simulink model "RAM_Design"  (R2025a)
settings: Solver=FixedStepDiscrete  StartTime=0.0  StopTime=10  FixedStep=1e-6  RelTol=1e-3
undefined symbols (not defined in the file): Bit_1, Bit_2, Bit_3, Bit_4, Bit_5, Bit_6, Bit_7, Bit_8
libraries: fl_lib x320, nesl_utility x136, simulink_extras x57
(part 1 of 5)
settings Model: PacingRate=0.050000  Creator=gerri  LastModifiedBy=gerri

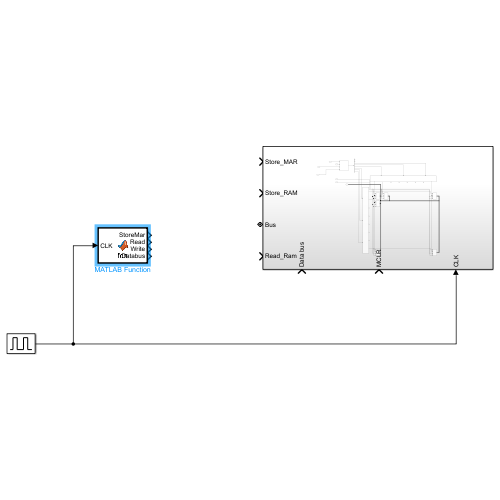
[thumbnail: Simulink's stored preview of the top-level diagram]
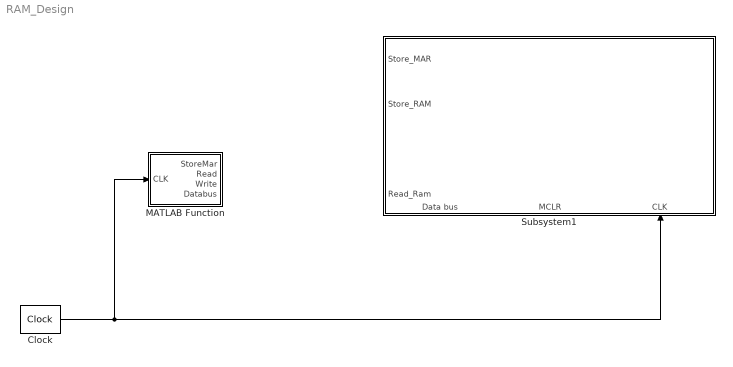
== system RAM_Design ==
  Clock : simulink_extras/Flip Flops/Clock  period=0.001
  MATLAB Function : MATLAB Function  TreatAsAtomicUnit=on
  Subsystem1 : Subsystem
      settings: PortSchema="{\"entries\":[{\"content\":{\"sides\":[{\"content\":{\"connectorIds\":[\"In1\",\"In2\",\"LConn1\",\"In3\"]},\"type\":\"ConnectorPlacement.EquallySpacedRectSide\",\"uuid\":\"fc099c56-c4b8-4508-a941-00bff1c84ffc\"},{\"content\":{\"side\":\"RIGHT\"},\"type\":\"ConnectorPlacement.EquallySpacedRectSide\",\"uuid\":\"202975a6-ae93-47c5-a757-f8e519a18074\"},{\"content\":{\"side\":\"TOP\"},\"type\":\"ConnectorPlacement.EquallySpacedRectSide\",\"uuid\":\"88b1988a-005b-4761-b740-e134c8683746\"},{\"content\":{\"connectorIds\":[\"In4\",\"In5\",\"In6\"],\"side\":\"BOTTOM\"},\"type\":\"ConnectorPlacement.EquallySpacedRectSide\",\"uuid\":\"5db4ec79-cfd7-4bc1-a90d-f6980e3bb618\"}]},\"type\":\"ConnectorPlacement.EquallySpacedConnector\",\"uuid\":\"bf959895-2947-4105-9e30-982428eecfc4\"}],\"packageUris\":[\"http://schema.mathworks.com/mf0/Connector/R2020b\"],\"version\":\"1.0\"}"
  wires:
  Clock/1 -> MATLAB Function/1(CLK), Subsystem1/6(CLK)

== system RAM_Design/Subsystem1 ==
  Store_MAR : Inport
  Store_RAM : Inport  Port=2
  Read_Ram : Inport  Port=3
  Data bus : Inport  Port=4
  MCLR : Inport  Port=5
  CLK : Inport  Port=6
  3*8_x : Subsystem
  3*8_y : Subsystem
  8Bit RAM 0 : Subsystem
  8Bit RAM 1 : Subsystem
  8Bit RAM 56 : Subsystem
  8Bit RAM 63 : Subsystem
  8Bit RAM 7 : Subsystem
  8Bit RAM 8 : Subsystem
  Demux : Demux  Outputs=8
  MAR : Subsystem
  Bus : PMIOPort  Side=Left
  wires:
  3*8_x/8(1/1/1) -> 8Bit RAM 7/1(x), 8Bit RAM 63/1(x)
  Demux/3 -> 3*8_y/3(Sel_C)
  3*8_x/1(0/0/0) -> 8Bit RAM 0/1(x), 8Bit RAM 8/1(x), 8Bit RAM 56/1(x)
  3*8_x/2(0/0/1) -> 8Bit RAM 1/1(x)
  3*8_y/1(0/0/0) -> 8Bit RAM 0/2(y), 8Bit RAM 1/2(y), 8Bit RAM 7/2(y)
  3*8_y/8(1/1/1) -> 8Bit RAM 63/2(y), 8Bit RAM 56/2(y)
  3*8_y/2(1/0/0) -> 8Bit RAM 8/2(y)
  Demux/4 -> 3*8_y/2(Sel_B)
  Demux/6 -> 3*8_x/1(Sel_A)
  Demux/7 -> 3*8_x/2(Sel_B)
  Demux/5 -> 3*8_y/1(Sel_A)
  MAR/1("Q Bus ") -> Demux/1
  Demux/8 -> 3*8_x/3(Sel_C)
  Store_RAM/1 -> 8Bit RAM 8/4(Store), 8Bit RAM 56/4(Store), 8Bit RAM 63/4(Store), 8Bit RAM 7/4(Store), 8Bit RAM 1/4(Store), 8Bit RAM 0/4(Store)
  CLK/1 -> MAR/3(CLK)
  Data bus/1 -> MAR/1(Data bus)
  Store_MAR/1 -> MAR/2(Store)
  MCLR/1 -> MAR/4(CLR)
  Read_Ram/1 -> 8Bit RAM 7/3(Enable), 8Bit RAM 1/3(Enable), 8Bit RAM 0/3(Enable), 8Bit RAM 56/3(Enable), 8Bit RAM 63/3(Enable), 8Bit RAM 8/3(Enable)
  connections:
  8Bit RAM 63/RConn1 -- 8Bit RAM 1/RConn1 -- 8Bit RAM 7/RConn1 -- 8Bit RAM 0/RConn1 -- Bus/RConn1 -- 8Bit RAM 8/RConn1 -- 8Bit RAM 56/RConn1

== system RAM_Design/Subsystem1/3*8_x ==
  note: A/B/C
  Sel_A : Inport
  Sel_B : Inport  Port=2
  Sel_C : Inport  Port=3
  AND{3..10} (8 alike) : Logic  Inputs=3  IconShape=distinctive  AllPortsSameDT=off  OutDataTypeStr=boolean
  NOT1 : Logic  Operator=NOT  IconShape=distinctive  AllPortsSameDT=off  OutDataTypeStr=boolean
  NOT2 : Logic  Operator=NOT  IconShape=distinctive  AllPortsSameDT=off  OutDataTypeStr=boolean
  NOT3 : Logic  Operator=NOT  IconShape=distinctive  AllPortsSameDT=off  OutDataTypeStr=boolean
  0/0/0 : Outport
  0/0/1 : Outport  Port=2
  0/1/0 : Outport  Port=3
  0/1/1 : Outport  Port=4
  1/0/0 : Outport  Port=5
  1/0/1 : Outport  Port=6
  1/1/0 : Outport  Port=7
  1/1/1 : Outport  Port=8
  wires:
  Sel_B/1 -> AND10/2, AND9/2, AND6/2, AND5/2, NOT2/1
  Sel_C/1 -> AND10/3, AND8/3, AND6/3, AND4/3, NOT3/1
  AND7/1 -> 1/0/0/1
  AND8/1 -> 1/0/1/1
  AND10/1 -> 1/1/1/1
  AND3/1 -> 0/0/0/1
  NOT1/1 -> AND6/1, AND5/1, AND4/1, AND3/1
  Sel_A/1 -> AND10/1, AND9/1, AND8/1, AND7/1, NOT1/1
  NOT3/1 -> AND9/3, AND7/3, AND5/3, AND3/3
  AND5/1 -> 0/1/0/1
  NOT2/1 -> AND4/2, AND7/2, AND8/2, AND3/2
  AND9/1 -> 1/1/0/1
  AND6/1 -> 0/1/1/1
  AND4/1 -> 0/0/1/1

== system RAM_Design/Subsystem1/3*8_y ==
  note: A/B/C
  Sel_A : Inport
  Sel_B : Inport  Port=2
  Sel_C : Inport  Port=3
  AND{3..10} (8 alike) : Logic  Inputs=3  IconShape=distinctive  AllPortsSameDT=off  OutDataTypeStr=boolean
  NOT1 : Logic  Operator=NOT  IconShape=distinctive  AllPortsSameDT=off  OutDataTypeStr=boolean
  NOT2 : Logic  Operator=NOT  IconShape=distinctive  AllPortsSameDT=off  OutDataTypeStr=boolean
  NOT3 : Logic  Operator=NOT  IconShape=distinctive  AllPortsSameDT=off  OutDataTypeStr=boolean
  0/0/0 : Outport
  1/0/0 : Outport  Port=2
  0/1/0 : Outport  Port=3
  1/1/0 : Outport  Port=4
  0/0/1 : Outport  Port=5
  1/0/1 : Outport  Port=6
  0/1/1 : Outport  Port=7
  1/1/1 : Outport  Port=8
  wires:
  Sel_B/1 -> AND10/2, AND9/2, AND6/2, AND5/2, NOT2/1
  Sel_C/1 -> AND10/3, AND8/3, AND6/3, AND4/3, NOT3/1
  AND7/1 -> 1/0/0/1
  AND8/1 -> 1/0/1/1
  AND10/1 -> 1/1/1/1
  AND3/1 -> 0/0/0/1
  NOT1/1 -> AND6/1, AND5/1, AND4/1, AND3/1
  Sel_A/1 -> AND10/1, AND9/1, AND8/1, AND7/1, NOT1/1
  NOT3/1 -> AND9/3, AND7/3, AND5/3, AND3/3
  AND5/1 -> 0/1/0/1
  NOT2/1 -> AND4/2, AND7/2, AND8/2, AND3/2
  AND9/1 -> 1/1/0/1
  AND6/1 -> 0/1/1/1
  AND4/1 -> 0/0/1/1

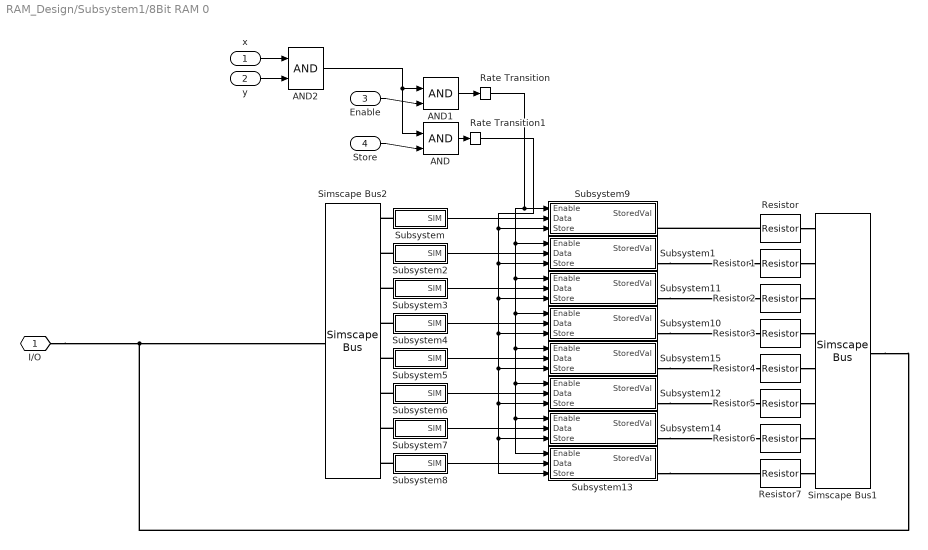
== system RAM_Design/Subsystem1/8Bit RAM 0 ==
  x : Inport
  y : Inport  Port=2
  Enable : Inport  Port=3
  Store : Inport  Port=4
  AND : Logic  IconShape=distinctive  AllPortsSameDT=off  OutDataTypeStr=boolean
  AND1 : Logic  IconShape=distinctive  AllPortsSameDT=off  OutDataTypeStr=boolean
  AND2 : Logic  IconShape=distinctive  AllPortsSameDT=off  OutDataTypeStr=boolean
  Rate Transition : RateTransition
  Rate Transition1 : RateTransition
  Resistor{,1..7} (8 alike) : fl_lib/Electrical/Electrical Elements/Resistor  R=1 Ohm  i_specify=off  i_priority=None  i=0 A  i_nominal_specify=off  i_nominal_value=1  i_nominal_unit=A  v_specify=off  v_priority=None  v=0 V  v_nominal_specify=off  v_nominal_value=1  v_nominal_unit=V
  Simscape Bus1 : SimscapeBus  HierarchyStrings=Bit_8;Bit_7;Bit_6;Bit_5;Bit_4;Bit_3;Bit_2;Bit_1
  Simscape Bus2 : SimscapeBus  HierarchyStrings=Bit_8;Bit_7;Bit_6;Bit_5;Bit_4;Bit_3;Bit_2;Bit_1
  Subsystem : Subsystem
  Subsystem1 : Subsystem
  Subsystem10 : Subsystem
  Subsystem11 : Subsystem
  Subsystem12 : Subsystem
  Subsystem13 : Subsystem
  Subsystem14 : Subsystem
  Subsystem15 : Subsystem
  Subsystem2 : Subsystem
  Subsystem3 : Subsystem
  Subsystem4 : Subsystem
  Subsystem5 : Subsystem
  Subsystem6 : Subsystem
  Subsystem7 : Subsystem
  Subsystem8 : Subsystem
  Subsystem9 : Subsystem
  I/O : PMIOPort  Side=Right
  wires:
  Enable/1 -> AND1/2
  Store/1 -> AND/2
  AND2/1 -> AND/1, AND1/1
  x/1 -> AND2/1
  y/1 -> AND2/2
  Subsystem/1(SIM) -> Subsystem9/2(Data)
  Subsystem2/1(SIM) -> Subsystem1/2(Data)
  Subsystem3/1(SIM) -> Subsystem11/2(Data)
  Subsystem4/1(SIM) -> Subsystem10/2(Data)
  Rate Transition1/1 -> Subsystem1/3(Store), Subsystem11/3(Store), Subsystem10/3(Store), Subsystem15/3(Store), Subsystem12/3(Store), Subsystem14/3(Store), Subsystem13/3(Store), Subsystem9/3(Store)
  AND1/1 -> Rate Transition/1
  Subsystem8/1(SIM) -> Subsystem13/2(Data)
  Subsystem7/1(SIM) -> Subsystem14/2(Data)
  Subsystem6/1(SIM) -> Subsystem12/2(Data)
  Subsystem5/1(SIM) -> Subsystem15/2(Data)
  Rate Transition/1 -> Subsystem1/1(Enable), Subsystem11/1(Enable), Subsystem10/1(Enable), Subsystem15/1(Enable), Subsystem12/1(Enable), Subsystem13/1(Enable), Subsystem14/1(Enable), Subsystem9/1(Enable)
  AND/1 -> Rate Transition1/1
  connections:
  I/O/RConn1 -- Simscape Bus1/RConn1 -- Simscape Bus2/RConn1
  Subsystem/LConn1 -- Simscape Bus2/LConn1
  Subsystem2/LConn1 -- Simscape Bus2/LConn2
  Subsystem4/LConn1 -- Simscape Bus2/LConn4
  Subsystem8/LConn1 -- Simscape Bus2/LConn8
  Subsystem6/LConn1 -- Simscape Bus2/LConn6
  Subsystem5/LConn1 -- Simscape Bus2/LConn5
  Subsystem7/LConn1 -- Simscape Bus2/LConn7
  Subsystem3/LConn1 -- Simscape Bus2/LConn3
  Resistor/RConn1 -- Simscape Bus1/LConn1
  Resistor/LConn1 -- Subsystem9/RConn1
  Subsystem1/RConn1 -- Resistor1/LConn1
  Resistor1/RConn1 -- Simscape Bus1/LConn2
  Subsystem10/RConn1 -- Resistor3/LConn1
  Subsystem11/RConn1 -- Resistor2/LConn1
  Resistor3/RConn1 -- Simscape Bus1/LConn4
  Resistor7/RConn1 -- Simscape Bus1/LConn8
  Resistor6/RConn1 -- Simscape Bus1/LConn7
  Resistor5/RConn1 -- Simscape Bus1/LConn6
  Resistor4/RConn1 -- Simscape Bus1/LConn5
  Resistor2/RConn1 -- Simscape Bus1/LConn3
  Subsystem15/RConn1 -- Resistor4/LConn1
  Subsystem12/RConn1 -- Resistor5/LConn1
  Subsystem14/RConn1 -- Resistor6/LConn1
  Subsystem13/RConn1 -- Resistor7/LConn1

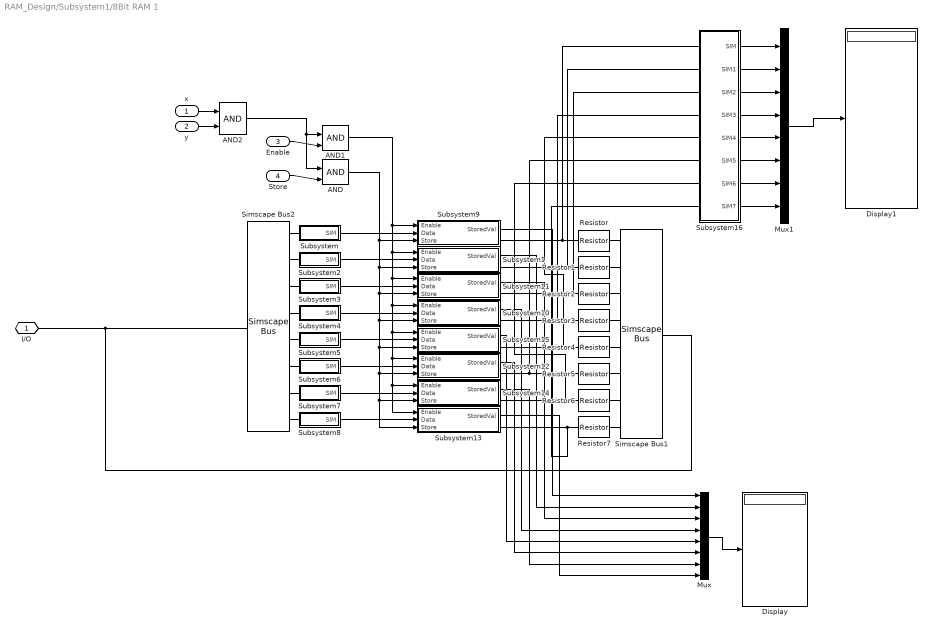
== system RAM_Design/Subsystem1/8Bit RAM 1 ==
  x : Inport
  y : Inport  Port=2
  Enable : Inport  Port=3
  Store : Inport  Port=4
  AND : Logic  IconShape=distinctive  AllPortsSameDT=off  OutDataTypeStr=boolean
  AND1 : Logic  IconShape=distinctive  AllPortsSameDT=off  OutDataTypeStr=boolean
  AND2 : Logic  IconShape=distinctive  AllPortsSameDT=off  OutDataTypeStr=boolean
  Display : Display
  Display1 : Display
  Mux : Mux  Inputs=8
  Mux1 : Mux  Inputs=8
  Resistor{,1..7} (8 alike) : fl_lib/Electrical/Electrical Elements/Resistor  R=1 Ohm  i_specify=off  i_priority=None  i=0 A  i_nominal_specify=off  i_nominal_value=1  i_nominal_unit=A  v_specify=off  v_priority=None  v=0 V  v_nominal_specify=off  v_nominal_value=1  v_nominal_unit=V
  Simscape Bus1 : SimscapeBus  HierarchyStrings=Bit_8;Bit_7;Bit_6;Bit_5;Bit_4;Bit_3;Bit_2;Bit_1
  Simscape Bus2 : SimscapeBus  HierarchyStrings=Bit_8;Bit_7;Bit_6;Bit_5;Bit_4;Bit_3;Bit_2;Bit_1
  Subsystem : Subsystem
  Subsystem1 : Subsystem
  Subsystem10 : Subsystem
  Subsystem11 : Subsystem
  Subsystem12 : Subsystem
  Subsystem13 : Subsystem
  Subsystem14 : Subsystem
  Subsystem15 : Subsystem
  Subsystem16 : Subsystem
  Subsystem2 : Subsystem
  Subsystem3 : Subsystem
  Subsystem4 : Subsystem
  Subsystem5 : Subsystem
  Subsystem6 : Subsystem
  Subsystem7 : Subsystem
  Subsystem8 : Subsystem
  Subsystem9 : Subsystem
  I/O : PMIOPort  Side=Right
  wires:
  Enable/1 -> AND1/2
  Store/1 -> AND/2
  AND2/1 -> AND/1, AND1/1
  x/1 -> AND2/1
  y/1 -> AND2/2
  Subsystem/1(SIM) -> Subsystem9/2(Data)
  Subsystem2/1(SIM) -> Subsystem1/2(Data)
  Subsystem3/1(SIM) -> Subsystem11/2(Data)
  Subsystem4/1(SIM) -> Subsystem10/2(Data)
  AND/1 -> Subsystem1/3(Store), Subsystem11/3(Store), Subsystem10/3(Store), Subsystem15/3(Store), Subsystem12/3(Store), Subsystem14/3(Store), Subsystem13/3(Store), Subsystem9/3(Store)
  AND1/1 -> Subsystem1/1(Enable), Subsystem11/1(Enable), Subsystem10/1(Enable), Subsystem15/1(Enable), Subsystem12/1(Enable), Subsystem13/1(Enable), Subsystem14/1(Enable), Subsystem9/1(Enable)
  Subsystem8/1(SIM) -> Subsystem13/2(Data)
  Subsystem7/1(SIM) -> Subsystem14/2(Data)
  Subsystem6/1(SIM) -> Subsystem12/2(Data)
  Subsystem5/1(SIM) -> Subsystem15/2(Data)
  Mux/1 -> Display/1
  Subsystem9/1(StoredVal) -> Mux/1
  Subsystem1/1(StoredVal) -> Mux/2
  Subsystem11/1(StoredVal) -> Mux/3
  Subsystem10/1(StoredVal) -> Mux/4
  Subsystem15/1(StoredVal) -> Mux/5
  Subsystem12/1(StoredVal) -> Mux/6
  Subsystem14/1(StoredVal) -> Mux/7
  Subsystem13/1(StoredVal) -> Mux/8
  Subsystem16/8(SIM7) -> Mux1/8
  Subsystem16/3(SIM2) -> Mux1/3
  Subsystem16/7(SIM6) -> Mux1/7
  Subsystem16/4(SIM3) -> Mux1/4
  Subsystem16/6(SIM5) -> Mux1/6
  Subsystem16/1(SIM) -> Mux1/1
  Subsystem16/5(SIM4) -> Mux1/5
  Subsystem16/2(SIM1) -> Mux1/2
  Mux1/1 -> Display1/1
  connections:
  I/O/RConn1 -- Simscape Bus1/RConn1 -- Simscape Bus2/RConn1
  Subsystem/LConn1 -- Simscape Bus2/LConn1
  Subsystem2/LConn1 -- Simscape Bus2/LConn2
  Subsystem4/LConn1 -- Simscape Bus2/LConn4
  Subsystem8/LConn1 -- Simscape Bus2/LConn8
  Subsystem6/LConn1 -- Simscape Bus2/LConn6
  Subsystem5/LConn1 -- Simscape Bus2/LConn5
  Subsystem7/LConn1 -- Simscape Bus2/LConn7
  Subsystem3/LConn1 -- Simscape Bus2/LConn3
  Resistor/RConn1 -- Simscape Bus1/LConn1
  Resistor/LConn1 -- Subsystem16/LConn1 -- Subsystem9/RConn1
  Resistor1/LConn1 -- Subsystem1/RConn1 -- Subsystem16/LConn2
  Resistor1/RConn1 -- Simscape Bus1/LConn2
  Resistor3/LConn1 -- Subsystem10/RConn1 -- Subsystem16/LConn4
  Resistor2/LConn1 -- Subsystem11/RConn1 -- Subsystem16/LConn3
  Resistor3/RConn1 -- Simscape Bus1/LConn4
  Resistor7/RConn1 -- Simscape Bus1/LConn8
  Resistor6/RConn1 -- Simscape Bus1/LConn7
  Resistor5/RConn1 -- Simscape Bus1/LConn6
  Resistor4/RConn1 -- Simscape Bus1/LConn5
  Resistor2/RConn1 -- Simscape Bus1/LConn3
  Resistor4/LConn1 -- Subsystem15/RConn1 -- Subsystem16/LConn5
  Resistor5/LConn1 -- Subsystem12/RConn1 -- Subsystem16/LConn6
  Resistor6/LConn1 -- Subsystem14/RConn1 -- Subsystem16/LConn7
  Resistor7/LConn1 -- Subsystem13/RConn1 -- Subsystem16/LConn8

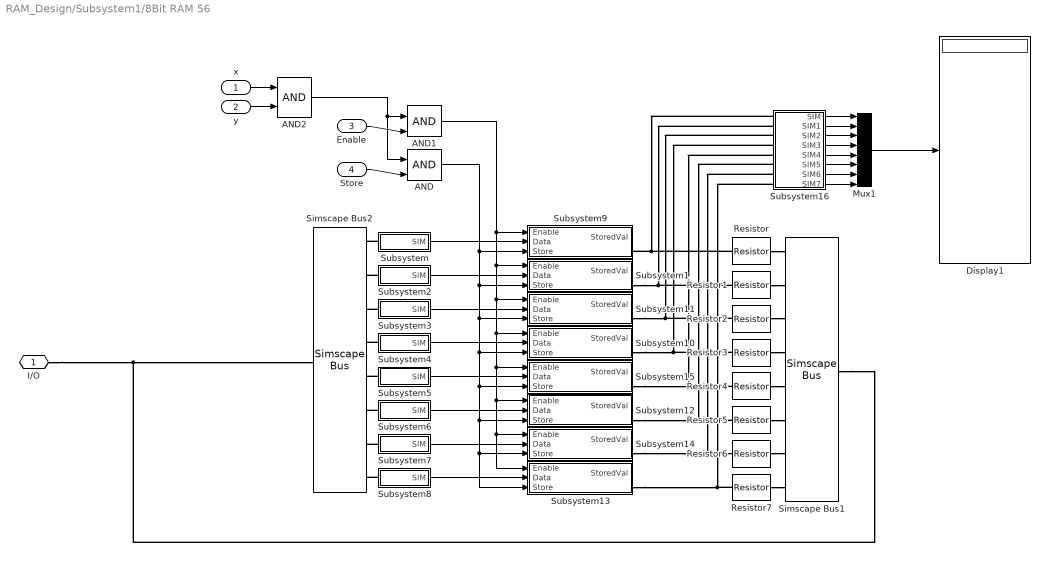
== system RAM_Design/Subsystem1/8Bit RAM 56 ==
  x : Inport
  y : Inport  Port=2
  Enable : Inport  Port=3
  Store : Inport  Port=4
  AND : Logic  IconShape=distinctive  AllPortsSameDT=off  OutDataTypeStr=boolean
  AND1 : Logic  IconShape=distinctive  AllPortsSameDT=off  OutDataTypeStr=boolean
  AND2 : Logic  IconShape=distinctive  AllPortsSameDT=off  OutDataTypeStr=boolean
  Display1 : Display
  Mux1 : Mux  Inputs=8
  Resistor{,1..7} (8 alike) : fl_lib/Electrical/Electrical Elements/Resistor  R=1 Ohm  i_specify=off  i_priority=None  i=0 A  i_nominal_specify=off  i_nominal_value=1  i_nominal_unit=A  v_specify=off  v_priority=None  v=0 V  v_nominal_specify=off  v_nominal_value=1  v_nominal_unit=V
  Simscape Bus1 : SimscapeBus  HierarchyStrings=Bit_8;Bit_7;Bit_6;Bit_5;Bit_4;Bit_3;Bit_2;Bit_1
  Simscape Bus2 : SimscapeBus  HierarchyStrings=Bit_8;Bit_7;Bit_6;Bit_5;Bit_4;Bit_3;Bit_2;Bit_1
  Subsystem : Subsystem
  Subsystem1 : Subsystem
  Subsystem10 : Subsystem
  Subsystem11 : Subsystem
  Subsystem12 : Subsystem
  Subsystem13 : Subsystem
  Subsystem14 : Subsystem
  Subsystem15 : Subsystem
  Subsystem16 : Subsystem
  Subsystem2 : Subsystem
  Subsystem3 : Subsystem
  Subsystem4 : Subsystem
  Subsystem5 : Subsystem
  Subsystem6 : Subsystem
  Subsystem7 : Subsystem
  Subsystem8 : Subsystem
  Subsystem9 : Subsystem
  I/O : PMIOPort  Side=Right
  wires:
  Enable/1 -> AND1/2
  Store/1 -> AND/2
  AND2/1 -> AND/1, AND1/1
  x/1 -> AND2/1
  y/1 -> AND2/2
  Subsystem/1(SIM) -> Subsystem9/2(Data)
  Subsystem2/1(SIM) -> Subsystem1/2(Data)
  Subsystem3/1(SIM) -> Subsystem11/2(Data)
  Subsystem4/1(SIM) -> Subsystem10/2(Data)
  AND/1 -> Subsystem1/3(Store), Subsystem11/3(Store), Subsystem10/3(Store), Subsystem15/3(Store), Subsystem12/3(Store), Subsystem14/3(Store), Subsystem13/3(Store), Subsystem9/3(Store)
  AND1/1 -> Subsystem1/1(Enable), Subsystem11/1(Enable), Subsystem10/1(Enable), Subsystem15/1(Enable), Subsystem12/1(Enable), Subsystem13/1(Enable), Subsystem14/1(Enable), Subsystem9/1(Enable)
  Subsystem8/1(SIM) -> Subsystem13/2(Data)
  Subsystem7/1(SIM) -> Subsystem14/2(Data)
  Subsystem6/1(SIM) -> Subsystem12/2(Data)
  Subsystem5/1(SIM) -> Subsystem15/2(Data)
  Subsystem16/8(SIM7) -> Mux1/8
  Subsystem16/3(SIM2) -> Mux1/3
  Subsystem16/7(SIM6) -> Mux1/7
  Subsystem16/4(SIM3) -> Mux1/4
  Subsystem16/6(SIM5) -> Mux1/6
  Subsystem16/1(SIM) -> Mux1/1
  Subsystem16/5(SIM4) -> Mux1/5
  Subsystem16/2(SIM1) -> Mux1/2
  Mux1/1 -> Display1/1
  connections:
  I/O/RConn1 -- Simscape Bus1/RConn1 -- Simscape Bus2/RConn1
  Subsystem/LConn1 -- Simscape Bus2/LConn1
  Subsystem2/LConn1 -- Simscape Bus2/LConn2
  Subsystem4/LConn1 -- Simscape Bus2/LConn4
  Subsystem8/LConn1 -- Simscape Bus2/LConn8
  Subsystem6/LConn1 -- Simscape Bus2/LConn6
  Subsystem5/LConn1 -- Simscape Bus2/LConn5
  Subsystem7/LConn1 -- Simscape Bus2/LConn7
  Subsystem3/LConn1 -- Simscape Bus2/LConn3
  Resistor/RConn1 -- Simscape Bus1/LConn1
  Subsystem16/LConn1 -- Resistor/LConn1 -- Subsystem9/RConn1
  Resistor1/LConn1 -- Subsystem1/RConn1 -- Subsystem16/LConn2
  Resistor1/RConn1 -- Simscape Bus1/LConn2
  Resistor3/LConn1 -- Subsystem10/RConn1 -- Subsystem16/LConn4
  Resistor2/LConn1 -- Subsystem11/RConn1 -- Subsystem16/LConn3
  Resistor3/RConn1 -- Simscape Bus1/LConn4
  Resistor7/RConn1 -- Simscape Bus1/LConn8
  Resistor6/RConn1 -- Simscape Bus1/LConn7
  Resistor5/RConn1 -- Simscape Bus1/LConn6
  Resistor4/RConn1 -- Simscape Bus1/LConn5
  Resistor2/RConn1 -- Simscape Bus1/LConn3
  Resistor4/LConn1 -- Subsystem15/RConn1 -- Subsystem16/LConn5
  Resistor5/LConn1 -- Subsystem12/RConn1 -- Subsystem16/LConn6
  Subsystem14/RConn1 -- Resistor6/LConn1 -- Subsystem16/LConn7
  Subsystem13/RConn1 -- Resistor7/LConn1 -- Subsystem16/LConn8

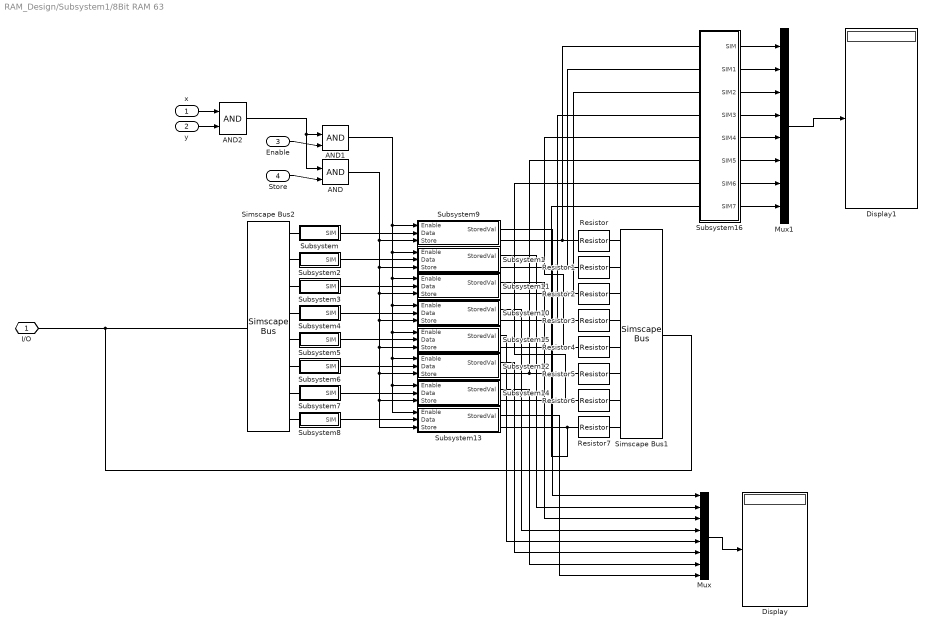
== system RAM_Design/Subsystem1/8Bit RAM 63 ==
  x : Inport
  y : Inport  Port=2
  Enable : Inport  Port=3
  Store : Inport  Port=4
  AND : Logic  IconShape=distinctive  AllPortsSameDT=off  OutDataTypeStr=boolean
  AND1 : Logic  IconShape=distinctive  AllPortsSameDT=off  OutDataTypeStr=boolean
  AND2 : Logic  IconShape=distinctive  AllPortsSameDT=off  OutDataTypeStr=boolean
  Display : Display
  Display1 : Display
  Mux : Mux  Inputs=8
  Mux1 : Mux  Inputs=8
  Resistor{,1..7} (8 alike) : fl_lib/Electrical/Electrical Elements/Resistor  R=1 Ohm  i_specify=off  i_priority=None  i=0 A  i_nominal_specify=off  i_nominal_value=1  i_nominal_unit=A  v_specify=off  v_priority=None  v=0 V  v_nominal_specify=off  v_nominal_value=1  v_nominal_unit=V
  Simscape Bus1 : SimscapeBus  HierarchyStrings=Bit_8;Bit_7;Bit_6;Bit_5;Bit_4;Bit_3;Bit_2;Bit_1
  Simscape Bus2 : SimscapeBus  HierarchyStrings=Bit_8;Bit_7;Bit_6;Bit_5;Bit_4;Bit_3;Bit_2;Bit_1
  Subsystem : Subsystem
  Subsystem1 : Subsystem
  Subsystem10 : Subsystem
  Subsystem11 : Subsystem
  Subsystem12 : Subsystem
  Subsystem13 : Subsystem
  Subsystem14 : Subsystem
  Subsystem15 : Subsystem
  Subsystem16 : Subsystem
  Subsystem2 : Subsystem
  Subsystem3 : Subsystem
  Subsystem4 : Subsystem
  Subsystem5 : Subsystem
  Subsystem6 : Subsystem
  Subsystem7 : Subsystem
  Subsystem8 : Subsystem
  Subsystem9 : Subsystem
  I/O : PMIOPort  Side=Right
  wires:
  Enable/1 -> AND1/2
  Store/1 -> AND/2
  AND2/1 -> AND/1, AND1/1
  x/1 -> AND2/1
  y/1 -> AND2/2
  Subsystem/1(SIM) -> Subsystem9/2(Data)
  Subsystem2/1(SIM) -> Subsystem1/2(Data)
  Subsystem3/1(SIM) -> Subsystem11/2(Data)
  Subsystem4/1(SIM) -> Subsystem10/2(Data)
  AND/1 -> Subsystem1/3(Store), Subsystem11/3(Store), Subsystem10/3(Store), Subsystem15/3(Store), Subsystem12/3(Store), Subsystem14/3(Store), Subsystem13/3(Store), Subsystem9/3(Store)
  AND1/1 -> Subsystem1/1(Enable), Subsystem11/1(Enable), Subsystem10/1(Enable), Subsystem15/1(Enable), Subsystem12/1(Enable), Subsystem13/1(Enable), Subsystem14/1(Enable), Subsystem9/1(Enable)
  Subsystem8/1(SIM) -> Subsystem13/2(Data)
  Subsystem7/1(SIM) -> Subsystem14/2(Data)
  Subsystem6/1(SIM) -> Subsystem12/2(Data)
  Subsystem5/1(SIM) -> Subsystem15/2(Data)
  Mux/1 -> Display/1
  Subsystem9/1(StoredVal) -> Mux/1
  Subsystem1/1(StoredVal) -> Mux/2
  Subsystem11/1(StoredVal) -> Mux/3
  Subsystem10/1(StoredVal) -> Mux/4
  Subsystem15/1(StoredVal) -> Mux/5
  Subsystem12/1(StoredVal) -> Mux/6
  Subsystem14/1(StoredVal) -> Mux/7
  Subsystem13/1(StoredVal) -> Mux/8
  Subsystem16/8(SIM7) -> Mux1/8
  Subsystem16/3(SIM2) -> Mux1/3
  Subsystem16/7(SIM6) -> Mux1/7
  Subsystem16/4(SIM3) -> Mux1/4
  Subsystem16/6(SIM5) -> Mux1/6
  Subsystem16/1(SIM) -> Mux1/1
  Subsystem16/5(SIM4) -> Mux1/5
  Subsystem16/2(SIM1) -> Mux1/2
  Mux1/1 -> Display1/1
  connections:
  I/O/RConn1 -- Simscape Bus1/RConn1 -- Simscape Bus2/RConn1
  Subsystem/LConn1 -- Simscape Bus2/LConn1
  Subsystem2/LConn1 -- Simscape Bus2/LConn2
  Subsystem4/LConn1 -- Simscape Bus2/LConn4
  Subsystem8/LConn1 -- Simscape Bus2/LConn8
  Subsystem6/LConn1 -- Simscape Bus2/LConn6
  Subsystem5/LConn1 -- Simscape Bus2/LConn5
  Subsystem7/LConn1 -- Simscape Bus2/LConn7
  Subsystem3/LConn1 -- Simscape Bus2/LConn3
  Resistor/RConn1 -- Simscape Bus1/LConn1
  Resistor/LConn1 -- Subsystem16/LConn1 -- Subsystem9/RConn1
  Resistor1/LConn1 -- Subsystem1/RConn1 -- Subsystem16/LConn2
  Resistor1/RConn1 -- Simscape Bus1/LConn2
  Resistor3/LConn1 -- Subsystem10/RConn1 -- Subsystem16/LConn4
  Resistor2/LConn1 -- Subsystem11/RConn1 -- Subsystem16/LConn3
  Resistor3/RConn1 -- Simscape Bus1/LConn4
  Resistor7/RConn1 -- Simscape Bus1/LConn8
  Resistor6/RConn1 -- Simscape Bus1/LConn7
  Resistor5/RConn1 -- Simscape Bus1/LConn6
  Resistor4/RConn1 -- Simscape Bus1/LConn5
  Resistor2/RConn1 -- Simscape Bus1/LConn3
  Resistor4/LConn1 -- Subsystem15/RConn1 -- Subsystem16/LConn5
  Resistor5/LConn1 -- Subsystem12/RConn1 -- Subsystem16/LConn6
  Resistor6/LConn1 -- Subsystem14/RConn1 -- Subsystem16/LConn7
  Resistor7/LConn1 -- Subsystem13/RConn1 -- Subsystem16/LConn8

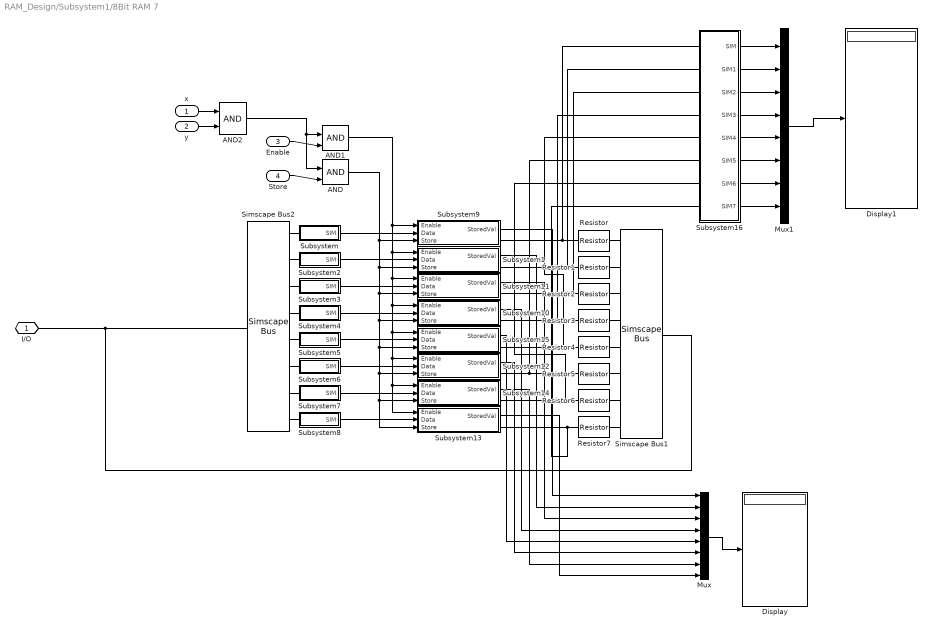
== system RAM_Design/Subsystem1/8Bit RAM 7 ==
  x : Inport
  y : Inport  Port=2
  Enable : Inport  Port=3
  Store : Inport  Port=4
  AND : Logic  IconShape=distinctive  AllPortsSameDT=off  OutDataTypeStr=boolean
  AND1 : Logic  IconShape=distinctive  AllPortsSameDT=off  OutDataTypeStr=boolean
  AND2 : Logic  IconShape=distinctive  AllPortsSameDT=off  OutDataTypeStr=boolean
  Display : Display
  Display1 : Display
  Mux : Mux  Inputs=8
  Mux1 : Mux  Inputs=8
  Resistor{,1..7} (8 alike) : fl_lib/Electrical/Electrical Elements/Resistor  R=1 Ohm  i_specify=off  i_priority=None  i=0 A  i_nominal_specify=off  i_nominal_value=1  i_nominal_unit=A  v_specify=off  v_priority=None  v=0 V  v_nominal_specify=off  v_nominal_value=1  v_nominal_unit=V
  Simscape Bus1 : SimscapeBus  HierarchyStrings=Bit_8;Bit_7;Bit_6;Bit_5;Bit_4;Bit_3;Bit_2;Bit_1
  Simscape Bus2 : SimscapeBus  HierarchyStrings=Bit_8;Bit_7;Bit_6;Bit_5;Bit_4;Bit_3;Bit_2;Bit_1
  Subsystem : Subsystem
  Subsystem1 : Subsystem
  Subsystem10 : Subsystem
  Subsystem11 : Subsystem
  Subsystem12 : Subsystem
  Subsystem13 : Subsystem
  Subsystem14 : Subsystem
  Subsystem15 : Subsystem
  Subsystem16 : Subsystem
  Subsystem2 : Subsystem
  Subsystem3 : Subsystem
  Subsystem4 : Subsystem
  Subsystem5 : Subsystem
  Subsystem6 : Subsystem
  Subsystem7 : Subsystem
  Subsystem8 : Subsystem
  Subsystem9 : Subsystem
  I/O : PMIOPort  Side=Right
  wires:
  Enable/1 -> AND1/2
  Store/1 -> AND/2
  AND2/1 -> AND/1, AND1/1
  x/1 -> AND2/1
  y/1 -> AND2/2
  Subsystem/1(SIM) -> Subsystem9/2(Data)
  Subsystem2/1(SIM) -> Subsystem1/2(Data)
  Subsystem3/1(SIM) -> Subsystem11/2(Data)
  Subsystem4/1(SIM) -> Subsystem10/2(Data)
  AND/1 -> Subsystem1/3(Store), Subsystem11/3(Store), Subsystem10/3(Store), Subsystem15/3(Store), Subsystem12/3(Store), Subsystem14/3(Store), Subsystem13/3(Store), Subsystem9/3(Store)
  AND1/1 -> Subsystem1/1(Enable), Subsystem11/1(Enable), Subsystem10/1(Enable), Subsystem15/1(Enable), Subsystem12/1(Enable), Subsystem13/1(Enable), Subsystem14/1(Enable), Subsystem9/1(Enable)
  Subsystem8/1(SIM) -> Subsystem13/2(Data)
  Subsystem7/1(SIM) -> Subsystem14/2(Data)
  Subsystem6/1(SIM) -> Subsystem12/2(Data)
  Subsystem5/1(SIM) -> Subsystem15/2(Data)
  Mux/1 -> Display/1
  Subsystem9/1(StoredVal) -> Mux/1
  Subsystem1/1(StoredVal) -> Mux/2
  Subsystem11/1(StoredVal) -> Mux/3
  Subsystem10/1(StoredVal) -> Mux/4
  Subsystem15/1(StoredVal) -> Mux/5
  Subsystem12/1(StoredVal) -> Mux/6
  Subsystem14/1(StoredVal) -> Mux/7
  Subsystem13/1(StoredVal) -> Mux/8
  Subsystem16/8(SIM7) -> Mux1/8
  Subsystem16/3(SIM2) -> Mux1/3
  Subsystem16/7(SIM6) -> Mux1/7
  Subsystem16/4(SIM3) -> Mux1/4
  Subsystem16/6(SIM5) -> Mux1/6
  Subsystem16/1(SIM) -> Mux1/1
  Subsystem16/5(SIM4) -> Mux1/5
  Subsystem16/2(SIM1) -> Mux1/2
  Mux1/1 -> Display1/1
  connections:
  I/O/RConn1 -- Simscape Bus1/RConn1 -- Simscape Bus2/RConn1
  Subsystem/LConn1 -- Simscape Bus2/LConn1
  Subsystem2/LConn1 -- Simscape Bus2/LConn2
  Subsystem4/LConn1 -- Simscape Bus2/LConn4
  Subsystem8/LConn1 -- Simscape Bus2/LConn8
  Subsystem6/LConn1 -- Simscape Bus2/LConn6
  Subsystem5/LConn1 -- Simscape Bus2/LConn5
  Subsystem7/LConn1 -- Simscape Bus2/LConn7
  Subsystem3/LConn1 -- Simscape Bus2/LConn3
  Resistor/RConn1 -- Simscape Bus1/LConn1
  Resistor/LConn1 -- Subsystem16/LConn1 -- Subsystem9/RConn1
  Resistor1/LConn1 -- Subsystem1/RConn1 -- Subsystem16/LConn2
  Resistor1/RConn1 -- Simscape Bus1/LConn2
  Resistor3/LConn1 -- Subsystem10/RConn1 -- Subsystem16/LConn4
  Resistor2/LConn1 -- Subsystem11/RConn1 -- Subsystem16/LConn3
  Resistor3/RConn1 -- Simscape Bus1/LConn4
  Resistor7/RConn1 -- Simscape Bus1/LConn8
  Resistor6/RConn1 -- Simscape Bus1/LConn7
  Resistor5/RConn1 -- Simscape Bus1/LConn6
  Resistor4/RConn1 -- Simscape Bus1/LConn5
  Resistor2/RConn1 -- Simscape Bus1/LConn3
  Resistor4/LConn1 -- Subsystem15/RConn1 -- Subsystem16/LConn5
  Resistor5/LConn1 -- Subsystem12/RConn1 -- Subsystem16/LConn6
  Resistor6/LConn1 -- Subsystem14/RConn1 -- Subsystem16/LConn7
  Resistor7/LConn1 -- Subsystem13/RConn1 -- Subsystem16/LConn8

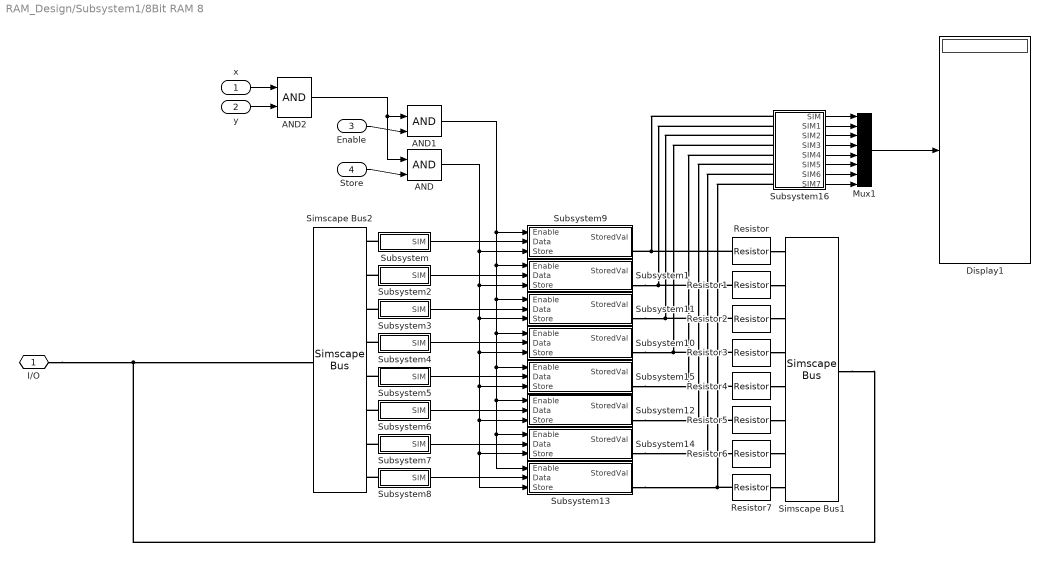
== system RAM_Design/Subsystem1/8Bit RAM 8 ==
  x : Inport
  y : Inport  Port=2
  Enable : Inport  Port=3
  Store : Inport  Port=4
  AND : Logic  IconShape=distinctive  AllPortsSameDT=off  OutDataTypeStr=boolean
  AND1 : Logic  IconShape=distinctive  AllPortsSameDT=off  OutDataTypeStr=boolean
  AND2 : Logic  IconShape=distinctive  AllPortsSameDT=off  OutDataTypeStr=boolean
  Display1 : Display
  Mux1 : Mux  Inputs=8
  Resistor{,1..7} (8 alike) : fl_lib/Electrical/Electrical Elements/Resistor  R=1 Ohm  i_specify=off  i_priority=None  i=0 A  i_nominal_specify=off  i_nominal_value=1  i_nominal_unit=A  v_specify=off  v_priority=None  v=0 V  v_nominal_specify=off  v_nominal_value=1  v_nominal_unit=V
  Simscape Bus1 : SimscapeBus  HierarchyStrings=Bit_8;Bit_7;Bit_6;Bit_5;Bit_4;Bit_3;Bit_2;Bit_1
  Simscape Bus2 : SimscapeBus  HierarchyStrings=Bit_8;Bit_7;Bit_6;Bit_5;Bit_4;Bit_3;Bit_2;Bit_1
  Subsystem : Subsystem
  Subsystem1 : Subsystem
  Subsystem10 : Subsystem
  Subsystem11 : Subsystem
  Subsystem12 : Subsystem
  Subsystem13 : Subsystem
  Subsystem14 : Subsystem
  Subsystem15 : Subsystem
  Subsystem16 : Subsystem
  Subsystem2 : Subsystem
  Subsystem3 : Subsystem
  Subsystem4 : Subsystem
  Subsystem5 : Subsystem
  Subsystem6 : Subsystem
  Subsystem7 : Subsystem
  Subsystem8 : Subsystem
  Subsystem9 : Subsystem
  I/O : PMIOPort  Side=Right
  wires:
  Enable/1 -> AND1/2
  Store/1 -> AND/2
  AND2/1 -> AND/1, AND1/1
  x/1 -> AND2/1
  y/1 -> AND2/2
  Subsystem/1(SIM) -> Subsystem9/2(Data)
  Subsystem2/1(SIM) -> Subsystem1/2(Data)
  Subsystem3/1(SIM) -> Subsystem11/2(Data)
  Subsystem4/1(SIM) -> Subsystem10/2(Data)
  AND/1 -> Subsystem1/3(Store), Subsystem11/3(Store), Subsystem10/3(Store), Subsystem15/3(Store), Subsystem12/3(Store), Subsystem14/3(Store), Subsystem13/3(Store), Subsystem9/3(Store)
  AND1/1 -> Subsystem1/1(Enable), Subsystem11/1(Enable), Subsystem10/1(Enable), Subsystem15/1(Enable), Subsystem12/1(Enable), Subsystem13/1(Enable), Subsystem14/1(Enable), Subsystem9/1(Enable)
  Subsystem8/1(SIM) -> Subsystem13/2(Data)
  Subsystem7/1(SIM) -> Subsystem14/2(Data)
  Subsystem6/1(SIM) -> Subsystem12/2(Data)
  Subsystem5/1(SIM) -> Subsystem15/2(Data)
  Subsystem16/8(SIM7) -> Mux1/8
  Subsystem16/3(SIM2) -> Mux1/3
  Subsystem16/7(SIM6) -> Mux1/7
  Subsystem16/4(SIM3) -> Mux1/4
  Subsystem16/6(SIM5) -> Mux1/6
  Subsystem16/1(SIM) -> Mux1/1
  Subsystem16/5(SIM4) -> Mux1/5
  Subsystem16/2(SIM1) -> Mux1/2
  Mux1/1 -> Display1/1
  connections:
  I/O/RConn1 -- Simscape Bus1/RConn1 -- Simscape Bus2/RConn1
  Subsystem/LConn1 -- Simscape Bus2/LConn1
  Subsystem2/LConn1 -- Simscape Bus2/LConn2
  Subsystem4/LConn1 -- Simscape Bus2/LConn4
  Subsystem8/LConn1 -- Simscape Bus2/LConn8
  Subsystem6/LConn1 -- Simscape Bus2/LConn6
  Subsystem5/LConn1 -- Simscape Bus2/LConn5
  Subsystem7/LConn1 -- Simscape Bus2/LConn7
  Subsystem3/LConn1 -- Simscape Bus2/LConn3
  Resistor/RConn1 -- Simscape Bus1/LConn1
  Subsystem16/LConn1 -- Resistor/LConn1 -- Subsystem9/RConn1
  Resistor1/LConn1 -- Subsystem1/RConn1 -- Subsystem16/LConn2
  Resistor1/RConn1 -- Simscape Bus1/LConn2
  Resistor3/LConn1 -- Subsystem10/RConn1 -- Subsystem16/LConn4
  Resistor2/LConn1 -- Subsystem11/RConn1 -- Subsystem16/LConn3
  Resistor3/RConn1 -- Simscape Bus1/LConn4
  Resistor7/RConn1 -- Simscape Bus1/LConn8
  Resistor6/RConn1 -- Simscape Bus1/LConn7
  Resistor5/RConn1 -- Simscape Bus1/LConn6
  Resistor4/RConn1 -- Simscape Bus1/LConn5
  Resistor2/RConn1 -- Simscape Bus1/LConn3
  Resistor4/LConn1 -- Subsystem15/RConn1 -- Subsystem16/LConn5
  Resistor5/LConn1 -- Subsystem12/RConn1 -- Subsystem16/LConn6
  Subsystem14/RConn1 -- Resistor6/LConn1 -- Subsystem16/LConn7
  Subsystem13/RConn1 -- Resistor7/LConn1 -- Subsystem16/LConn8

== system RAM_Design/Subsystem1/MAR ==
  Data bus : Inport
  Store : Inport  Port=2
  CLK : Inport  Port=3
  CLR : Inport  Port=4
  Demux : Demux  Outputs=8
  Mux : Mux  Inputs=8
  Subsystem1 : Subsystem
  Subsystem2 : Subsystem
  Subsystem3 : Subsystem
  Subsystem4 : Subsystem
  Subsystem5 : Subsystem
  Subsystem6 : Subsystem
  Subsystem7 : Subsystem
  Subsystem8 : Subsystem
  "Q Bus " : Outport
  wires:
  Demux/4 -> Subsystem2/1(Data)
  Mux/1 -> "Q Bus "/1
  Demux/2 -> Subsystem1/1(Data)
  Data bus/1 -> Demux/1
  Subsystem6/1(Q) -> Mux/8
  Store/1 -> Subsystem1/2(Store), Subsystem4/2(Store), Subsystem2/2(Store), Subsystem7/2(Store), Subsystem5/2(Store), Subsystem6/2(Store), Subsystem8/2(Store), Subsystem3/2(Store)
  Demux/5 -> Subsystem7/1(Data)
  Demux/7 -> Subsystem8/1(Data)
  Demux/3 -> Subsystem4/1(Data)
  Subsystem7/1(Q) -> Mux/5
  Demux/6 -> Subsystem5/1(Data)
  Subsystem1/1(Q) -> Mux/2
  Demux/1 -> Subsystem3/1(Data)
  Subsystem3/1(Q) -> Mux/1
  Demux/8 -> Subsystem6/1(Data)
  Subsystem8/1(Q) -> Mux/7
  Subsystem2/1(Q) -> Mux/4
  Subsystem4/1(Q) -> Mux/3
  Subsystem5/1(Q) -> Mux/6
  CLK/1 -> Subsystem1/3(Clock), Subsystem4/3(Clock), Subsystem2/3(Clock), Subsystem7/3(Clock), Subsystem5/3(Clock), Subsystem6/3(Clock), Subsystem8/3(Clock), Subsystem3/3(Clock)
  CLR/1 -> Subsystem8/4(Clear), Subsystem5/4(Clear), Subsystem7/4(Clear), Subsystem2/4(Clear), Subsystem4/4(Clear), Subsystem1/4(Clear), Subsystem3/4(Clear), Subsystem6/4(Clear)

== system RAM_Design/Subsystem1/8Bit RAM 0/Subsystem ==
  Cast To Boolean : DataTypeConversion  OutDataTypeStr=boolean  SaturateOnIntegerOverflow=off  RndMeth=Floor
  Delay One Step : Delay  DelayLength=1
  Electrical Reference : fl_lib/Electrical/Electrical Elements/Electrical Reference
  Gain : Gain  Gain=0.2
  PS-Simulink Converter : nesl_utility/PS-Simulink Converter  PhysicalDomain=network_engine_domain  SubClassName=ps_output  LeftPortType=input  RightPortType=output  PseudoPeriodic=off  Frequencies=[]  VectorFormat=inherit  Unit=inherit  AffineConversion=off
  Voltage Sensor : fl_lib/Electrical/Electrical Sensors/Voltage Sensor
  PS : PMIOPort  Side=Left
  SIM : Outport
  wires:
  PS-Simulink Converter/1 -> Gain/1
  Cast To Boolean/1 -> Delay One Step/1
  Gain/1 -> Cast To Boolean/1
  Delay One Step/1 -> SIM/1
  connections:
  PS/RConn1 -- Voltage Sensor/LConn1
  Electrical Reference/LConn1 -- Voltage Sensor/RConn2
  PS-Simulink Converter/LConn1 -- Voltage Sensor/RConn1

== system RAM_Design/Subsystem1/8Bit RAM 0/Subsystem1 ==
  Enable : Inport
  Data : Inport  Port=2
  Store : Inport  Port=3
  AND : Logic  IconShape=distinctive  AllPortsSameDT=off  OutDataTypeStr=boolean
  Cast To Double : DataTypeConversion  OutDataTypeStr=double  SaturateOnIntegerOverflow=off  RndMeth=Floor
  Controlled Voltage Source : fl_lib/Electrical/Electrical Sources/Controlled Voltage Source
  D Latch : simulink_extras/Flip Flops/D Latch
  Delay One Step : Delay  DelayLength=1  SampleTime=1e-6
  Electrical Reference : fl_lib/Electrical/Electrical Elements/Electrical Reference
  Gain : Gain  Gain=5
  Simulink-PS Converter : nesl_utility/Simulink-PS Converter  PhysicalDomain=network_engine_domain  SubClassName=ps_input  LeftPortType=input  RightPortType=output  PseudoPeriodic=off  Frequencies=[]  NoiseDistribution=none  NoiseParameters=[]  Unit=1  AffineConversion=off  FilteringAndDerivatives=provide  SimscapeFilterOrder=1  InputFilterTimeConstant=0.001  UdotUserProvided=0
  Q : PMIOPort  Side=Right
  StoredVal : Outport
  wires:
  AND/1 -> Delay One Step/1
  Store/1 -> D Latch/2
  Gain/1 -> Simulink-PS Converter/1
  D Latch/1 -> StoredVal/1, AND/1
  Cast To Double/1 -> Gain/1
  Enable/1 -> AND/2
  Data/1 -> D Latch/1
  Delay One Step/1 -> Cast To Double/1
  connections:
  Controlled Voltage Source/RConn1 -- Simulink-PS Converter/RConn1
  Electrical Reference/LConn1 -- Controlled Voltage Source/RConn2
  Controlled Voltage Source/LConn1 -- Q/RConn1

== system RAM_Design/Subsystem1/8Bit RAM 0/Subsystem10 ==
  Enable : Inport
  Data : Inport  Port=2
  Store : Inport  Port=3
  AND : Logic  IconShape=distinctive  AllPortsSameDT=off  OutDataTypeStr=boolean
  Cast To Double : DataTypeConversion  OutDataTypeStr=double  SaturateOnIntegerOverflow=off  RndMeth=Floor
  Controlled Voltage Source : fl_lib/Electrical/Electrical Sources/Controlled Voltage Source
  D Latch : simulink_extras/Flip Flops/D Latch
  Delay One Step : Delay  DelayLength=1
  Electrical Reference : fl_lib/Electrical/Electrical Elements/Electrical Reference
  Gain : Gain  Gain=5
  Simulink-PS Converter : nesl_utility/Simulink-PS Converter  PhysicalDomain=network_engine_domain  SubClassName=ps_input  LeftPortType=input  RightPortType=output  PseudoPeriodic=off  Frequencies=[]  NoiseDistribution=none  NoiseParameters=[]  Unit=1  AffineConversion=off  FilteringAndDerivatives=provide  SimscapeFilterOrder=1  InputFilterTimeConstant=0.001  UdotUserProvided=0
  Q : PMIOPort  Side=Right
  StoredVal : Outport
  wires:
  AND/1 -> Delay One Step/1
  Store/1 -> D Latch/2
  Gain/1 -> Simulink-PS Converter/1
  D Latch/1 -> StoredVal/1, AND/1
  Cast To Double/1 -> Gain/1
  Enable/1 -> AND/2
  Data/1 -> D Latch/1
  Delay One Step/1 -> Cast To Double/1
  connections:
  Controlled Voltage Source/RConn1 -- Simulink-PS Converter/RConn1
  Electrical Reference/LConn1 -- Controlled Voltage Source/RConn2
  Controlled Voltage Source/LConn1 -- Q/RConn1

== system RAM_Design/Subsystem1/8Bit RAM 0/Subsystem11 ==
  Enable : Inport
  Data : Inport  Port=2
  Store : Inport  Port=3
  AND : Logic  IconShape=distinctive  AllPortsSameDT=off  OutDataTypeStr=boolean
  Cast To Double : DataTypeConversion  OutDataTypeStr=double  SaturateOnIntegerOverflow=off  RndMeth=Floor
  Controlled Voltage Source : fl_lib/Electrical/Electrical Sources/Controlled Voltage Source
  D Latch : simulink_extras/Flip Flops/D Latch
  Delay One Step : Delay  DelayLength=1
  Electrical Reference : fl_lib/Electrical/Electrical Elements/Electrical Reference
  Gain : Gain  Gain=5
  Simulink-PS Converter : nesl_utility/Simulink-PS Converter  PhysicalDomain=network_engine_domain  SubClassName=ps_input  LeftPortType=input  RightPortType=output  PseudoPeriodic=off  Frequencies=[]  NoiseDistribution=none  NoiseParameters=[]  Unit=1  AffineConversion=off  FilteringAndDerivatives=provide  SimscapeFilterOrder=1  InputFilterTimeConstant=0.001  UdotUserProvided=0
  Q : PMIOPort  Side=Right
  StoredVal : Outport
  wires:
  AND/1 -> Delay One Step/1
  Store/1 -> D Latch/2
  Gain/1 -> Simulink-PS Converter/1
  D Latch/1 -> StoredVal/1, AND/1
  Cast To Double/1 -> Gain/1
  Enable/1 -> AND/2
  Data/1 -> D Latch/1
  Delay One Step/1 -> Cast To Double/1
  connections:
  Controlled Voltage Source/RConn1 -- Simulink-PS Converter/RConn1
  Electrical Reference/LConn1 -- Controlled Voltage Source/RConn2
  Controlled Voltage Source/LConn1 -- Q/RConn1

== system RAM_Design/Subsystem1/8Bit RAM 0/Subsystem12 ==
  Enable : Inport
  Data : Inport  Port=2
  Store : Inport  Port=3
  AND : Logic  IconShape=distinctive  AllPortsSameDT=off  OutDataTypeStr=boolean
  Cast To Double : DataTypeConversion  OutDataTypeStr=double  SaturateOnIntegerOverflow=off  RndMeth=Floor
  Controlled Voltage Source : fl_lib/Electrical/Electrical Sources/Controlled Voltage Source
  D Latch : simulink_extras/Flip Flops/D Latch
  Delay One Step : Delay  DelayLength=1
  Electrical Reference : fl_lib/Electrical/Electrical Elements/Electrical Reference
  Gain : Gain  Gain=5
  Simulink-PS Converter : nesl_utility/Simulink-PS Converter  PhysicalDomain=network_engine_domain  SubClassName=ps_input  LeftPortType=input  RightPortType=output  PseudoPeriodic=off  Frequencies=[]  NoiseDistribution=none  NoiseParameters=[]  Unit=1  AffineConversion=off  FilteringAndDerivatives=provide  SimscapeFilterOrder=1  InputFilterTimeConstant=0.001  UdotUserProvided=0
  Q : PMIOPort  Side=Right
  StoredVal : Outport
  wires:
  AND/1 -> Delay One Step/1
  Store/1 -> D Latch/2
  Gain/1 -> Simulink-PS Converter/1
  D Latch/1 -> StoredVal/1, AND/1
  Cast To Double/1 -> Gain/1
  Enable/1 -> AND/2
  Data/1 -> D Latch/1
  Delay One Step/1 -> Cast To Double/1
  connections:
  Controlled Voltage Source/RConn1 -- Simulink-PS Converter/RConn1
  Electrical Reference/LConn1 -- Controlled Voltage Source/RConn2
  Controlled Voltage Source/LConn1 -- Q/RConn1

== system RAM_Design/Subsystem1/8Bit RAM 0/Subsystem13 ==
  Enable : Inport
  Data : Inport  Port=2
  Store : Inport  Port=3
  AND : Logic  IconShape=distinctive  AllPortsSameDT=off  OutDataTypeStr=boolean
  Cast To Double : DataTypeConversion  OutDataTypeStr=double  SaturateOnIntegerOverflow=off  RndMeth=Floor
  Controlled Voltage Source : fl_lib/Electrical/Electrical Sources/Controlled Voltage Source
  D Latch : simulink_extras/Flip Flops/D Latch
  Delay One Step : Delay  DelayLength=1
  Electrical Reference : fl_lib/Electrical/Electrical Elements/Electrical Reference
  Gain : Gain  Gain=5
  Simulink-PS Converter : nesl_utility/Simulink-PS Converter  PhysicalDomain=network_engine_domain  SubClassName=ps_input  LeftPortType=input  RightPortType=output  PseudoPeriodic=off  Frequencies=[]  NoiseDistribution=none  NoiseParameters=[]  Unit=1  AffineConversion=off  FilteringAndDerivatives=provide  SimscapeFilterOrder=1  InputFilterTimeConstant=0.001  UdotUserProvided=0
  Q : PMIOPort  Side=Right
  StoredVal : Outport
  wires:
  AND/1 -> Delay One Step/1
  Store/1 -> D Latch/2
  Gain/1 -> Simulink-PS Converter/1
  D Latch/1 -> StoredVal/1, AND/1
  Cast To Double/1 -> Gain/1
  Enable/1 -> AND/2
  Data/1 -> D Latch/1
  Delay One Step/1 -> Cast To Double/1
  connections:
  Controlled Voltage Source/RConn1 -- Simulink-PS Converter/RConn1
  Electrical Reference/LConn1 -- Controlled Voltage Source/RConn2
  Controlled Voltage Source/LConn1 -- Q/RConn1

== system RAM_Design/Subsystem1/8Bit RAM 0/Subsystem14 ==
  Enable : Inport
  Data : Inport  Port=2
  Store : Inport  Port=3
  AND : Logic  IconShape=distinctive  AllPortsSameDT=off  OutDataTypeStr=boolean
  Cast To Double : DataTypeConversion  OutDataTypeStr=double  SaturateOnIntegerOverflow=off  RndMeth=Floor
  Controlled Voltage Source : fl_lib/Electrical/Electrical Sources/Controlled Voltage Source
  D Latch : simulink_extras/Flip Flops/D Latch
  Delay One Step : Delay  DelayLength=1
  Electrical Reference : fl_lib/Electrical/Electrical Elements/Electrical Reference
  Gain : Gain  Gain=5
  Simulink-PS Converter : nesl_utility/Simulink-PS Converter  PhysicalDomain=network_engine_domain  SubClassName=ps_input  LeftPortType=input  RightPortType=output  PseudoPeriodic=off  Frequencies=[]  NoiseDistribution=none  NoiseParameters=[]  Unit=1  AffineConversion=off  FilteringAndDerivatives=provide  SimscapeFilterOrder=1  InputFilterTimeConstant=0.001  UdotUserProvided=0
  Q : PMIOPort  Side=Right
  StoredVal : Outport
  wires:
  AND/1 -> Delay One Step/1
  Store/1 -> D Latch/2
  Gain/1 -> Simulink-PS Converter/1
  D Latch/1 -> StoredVal/1, AND/1
  Cast To Double/1 -> Gain/1
  Enable/1 -> AND/2
  Data/1 -> D Latch/1
  Delay One Step/1 -> Cast To Double/1
  connections:
  Controlled Voltage Source/RConn1 -- Simulink-PS Converter/RConn1
  Electrical Reference/LConn1 -- Controlled Voltage Source/RConn2
  Controlled Voltage Source/LConn1 -- Q/RConn1

== system RAM_Design/Subsystem1/8Bit RAM 0/Subsystem15 ==
  Enable : Inport
  Data : Inport  Port=2
  Store : Inport  Port=3
  AND : Logic  IconShape=distinctive  AllPortsSameDT=off  OutDataTypeStr=boolean
  Cast To Double : DataTypeConversion  OutDataTypeStr=double  SaturateOnIntegerOverflow=off  RndMeth=Floor
  Controlled Voltage Source : fl_lib/Electrical/Electrical Sources/Controlled Voltage Source
  D Latch : simulink_extras/Flip Flops/D Latch
  Delay One Step : Delay  DelayLength=1
  Electrical Reference : fl_lib/Electrical/Electrical Elements/Electrical Reference
  Gain : Gain  Gain=5
  Simulink-PS Converter : nesl_utility/Simulink-PS Converter  PhysicalDomain=network_engine_domain  SubClassName=ps_input  LeftPortType=input  RightPortType=output  PseudoPeriodic=off  Frequencies=[]  NoiseDistribution=none  NoiseParameters=[]  Unit=1  AffineConversion=off  FilteringAndDerivatives=provide  SimscapeFilterOrder=1  InputFilterTimeConstant=0.001  UdotUserProvided=0
  Q : PMIOPort  Side=Right
  StoredVal : Outport
  wires:
  AND/1 -> Delay One Step/1
  Store/1 -> D Latch/2
  Gain/1 -> Simulink-PS Converter/1
  D Latch/1 -> StoredVal/1, AND/1
  Cast To Double/1 -> Gain/1
  Enable/1 -> AND/2
  Data/1 -> D Latch/1
  Delay One Step/1 -> Cast To Double/1
  connections:
  Controlled Voltage Source/RConn1 -- Simulink-PS Converter/RConn1
  Electrical Reference/LConn1 -- Controlled Voltage Source/RConn2
  Controlled Voltage Source/LConn1 -- Q/RConn1

== system RAM_Design/Subsystem1/8Bit RAM 0/Subsystem2 ==
  Cast To Boolean : DataTypeConversion  OutDataTypeStr=boolean  SaturateOnIntegerOverflow=off  RndMeth=Floor
  Delay One Step : Delay  DelayLength=1
  Electrical Reference : fl_lib/Electrical/Electrical Elements/Electrical Reference
  Gain : Gain  Gain=0.2
  PS-Simulink Converter : nesl_utility/PS-Simulink Converter  PhysicalDomain=network_engine_domain  SubClassName=ps_output  LeftPortType=input  RightPortType=output  PseudoPeriodic=off  Frequencies=[]  VectorFormat=inherit  Unit=inherit  AffineConversion=off
  Voltage Sensor : fl_lib/Electrical/Electrical Sensors/Voltage Sensor
  PS : PMIOPort  Side=Left
  SIM : Outport
  wires:
  PS-Simulink Converter/1 -> Gain/1
  Cast To Boolean/1 -> Delay One Step/1
  Gain/1 -> Cast To Boolean/1
  Delay One Step/1 -> SIM/1
  connections:
  PS/RConn1 -- Voltage Sensor/LConn1
  Electrical Reference/LConn1 -- Voltage Sensor/RConn2
  PS-Simulink Converter/LConn1 -- Voltage Sensor/RConn1

== system RAM_Design/Subsystem1/8Bit RAM 0/Subsystem3 ==
  Cast To Boolean : DataTypeConversion  OutDataTypeStr=boolean  SaturateOnIntegerOverflow=off  RndMeth=Floor
  Delay One Step : Delay  DelayLength=1
  Electrical Reference : fl_lib/Electrical/Electrical Elements/Electrical Reference
  Gain : Gain  Gain=0.2
  PS-Simulink Converter : nesl_utility/PS-Simulink Converter  PhysicalDomain=network_engine_domain  SubClassName=ps_output  LeftPortType=input  RightPortType=output  PseudoPeriodic=off  Frequencies=[]  VectorFormat=inherit  Unit=inherit  AffineConversion=off
  Voltage Sensor : fl_lib/Electrical/Electrical Sensors/Voltage Sensor
  PS : PMIOPort  Side=Left
  SIM : Outport
  wires:
  PS-Simulink Converter/1 -> Gain/1
  Cast To Boolean/1 -> Delay One Step/1
  Gain/1 -> Cast To Boolean/1
  Delay One Step/1 -> SIM/1
  connections:
  PS/RConn1 -- Voltage Sensor/LConn1
  Electrical Reference/LConn1 -- Voltage Sensor/RConn2
  PS-Simulink Converter/LConn1 -- Voltage Sensor/RConn1

== system RAM_Design/Subsystem1/8Bit RAM 0/Subsystem4 ==
  Cast To Boolean : DataTypeConversion  OutDataTypeStr=boolean  SaturateOnIntegerOverflow=off  RndMeth=Floor
  Delay One Step : Delay  DelayLength=1
  Electrical Reference : fl_lib/Electrical/Electrical Elements/Electrical Reference
  Gain : Gain  Gain=0.2
  PS-Simulink Converter : nesl_utility/PS-Simulink Converter  PhysicalDomain=network_engine_domain  SubClassName=ps_output  LeftPortType=input  RightPortType=output  PseudoPeriodic=off  Frequencies=[]  VectorFormat=inherit  Unit=inherit  AffineConversion=off
  Voltage Sensor : fl_lib/Electrical/Electrical Sensors/Voltage Sensor
  PS : PMIOPort  Side=Left
  SIM : Outport
  wires:
  PS-Simulink Converter/1 -> Gain/1
  Cast To Boolean/1 -> Delay One Step/1
  Gain/1 -> Cast To Boolean/1
  Delay One Step/1 -> SIM/1
  connections:
  PS/RConn1 -- Voltage Sensor/LConn1
  Electrical Reference/LConn1 -- Voltage Sensor/RConn2
  PS-Simulink Converter/LConn1 -- Voltage Sensor/RConn1

== system RAM_Design/Subsystem1/8Bit RAM 0/Subsystem5 ==
  Cast To Boolean : DataTypeConversion  OutDataTypeStr=boolean  SaturateOnIntegerOverflow=off  RndMeth=Floor
  Delay One Step : Delay  DelayLength=1
  Electrical Reference : fl_lib/Electrical/Electrical Elements/Electrical Reference
  Gain : Gain  Gain=0.2
  PS-Simulink Converter : nesl_utility/PS-Simulink Converter  PhysicalDomain=network_engine_domain  SubClassName=ps_output  LeftPortType=input  RightPortType=output  PseudoPeriodic=off  Frequencies=[]  VectorFormat=inherit  Unit=inherit  AffineConversion=off
  Voltage Sensor : fl_lib/Electrical/Electrical Sensors/Voltage Sensor
  PS : PMIOPort  Side=Left
  SIM : Outport
  wires:
  PS-Simulink Converter/1 -> Gain/1
  Cast To Boolean/1 -> Delay One Step/1
  Gain/1 -> Cast To Boolean/1
  Delay One Step/1 -> SIM/1
  connections:
  PS/RConn1 -- Voltage Sensor/LConn1
  Electrical Reference/LConn1 -- Voltage Sensor/RConn2
  PS-Simulink Converter/LConn1 -- Voltage Sensor/RConn1

== system RAM_Design/Subsystem1/8Bit RAM 0/Subsystem6 ==
  Cast To Boolean : DataTypeConversion  OutDataTypeStr=boolean  SaturateOnIntegerOverflow=off  RndMeth=Floor
  Delay One Step : Delay  DelayLength=1
  Electrical Reference : fl_lib/Electrical/Electrical Elements/Electrical Reference
  Gain : Gain  Gain=0.2
  PS-Simulink Converter : nesl_utility/PS-Simulink Converter  PhysicalDomain=network_engine_domain  SubClassName=ps_output  LeftPortType=input  RightPortType=output  PseudoPeriodic=off  Frequencies=[]  VectorFormat=inherit  Unit=inherit  AffineConversion=off
  Voltage Sensor : fl_lib/Electrical/Electrical Sensors/Voltage Sensor
  PS : PMIOPort  Side=Left
  SIM : Outport
  wires:
  PS-Simulink Converter/1 -> Gain/1
  Cast To Boolean/1 -> Delay One Step/1
  Gain/1 -> Cast To Boolean/1
  Delay One Step/1 -> SIM/1
  connections:
  PS/RConn1 -- Voltage Sensor/LConn1
  Electrical Reference/LConn1 -- Voltage Sensor/RConn2
  PS-Simulink Converter/LConn1 -- Voltage Sensor/RConn1

== system RAM_Design/Subsystem1/8Bit RAM 0/Subsystem7 ==
  Cast To Boolean : DataTypeConversion  OutDataTypeStr=boolean  SaturateOnIntegerOverflow=off  RndMeth=Floor
  Delay One Step : Delay  DelayLength=1
  Electrical Reference : fl_lib/Electrical/Electrical Elements/Electrical Reference
  Gain : Gain  Gain=0.2
  PS-Simulink Converter : nesl_utility/PS-Simulink Converter  PhysicalDomain=network_engine_domain  SubClassName=ps_output  LeftPortType=input  RightPortType=output  PseudoPeriodic=off  Frequencies=[]  VectorFormat=inherit  Unit=inherit  AffineConversion=off
  Voltage Sensor : fl_lib/Electrical/Electrical Sensors/Voltage Sensor
  PS : PMIOPort  Side=Left
  SIM : Outport
  wires:
  PS-Simulink Converter/1 -> Gain/1
  Cast To Boolean/1 -> Delay One Step/1
  Gain/1 -> Cast To Boolean/1
  Delay One Step/1 -> SIM/1
  connections:
  PS/RConn1 -- Voltage Sensor/LConn1
  Electrical Reference/LConn1 -- Voltage Sensor/RConn2
  PS-Simulink Converter/LConn1 -- Voltage Sensor/RConn1

== system RAM_Design/Subsystem1/8Bit RAM 0/Subsystem8 ==
  Cast To Boolean : DataTypeConversion  OutDataTypeStr=boolean  SaturateOnIntegerOverflow=off  RndMeth=Floor
  Delay One Step : Delay  DelayLength=1
  Electrical Reference : fl_lib/Electrical/Electrical Elements/Electrical Reference
  Gain : Gain  Gain=0.2
  PS-Simulink Converter : nesl_utility/PS-Simulink Converter  PhysicalDomain=network_engine_domain  SubClassName=ps_output  LeftPortType=input  RightPortType=output  PseudoPeriodic=off  Frequencies=[]  VectorFormat=inherit  Unit=inherit  AffineConversion=off
  Voltage Sensor : fl_lib/Electrical/Electrical Sensors/Voltage Sensor
  PS : PMIOPort  Side=Left
  SIM : Outport
  wires:
  PS-Simulink Converter/1 -> Gain/1
  Cast To Boolean/1 -> Delay One Step/1
  Gain/1 -> Cast To Boolean/1
  Delay One Step/1 -> SIM/1
  connections:
  PS/RConn1 -- Voltage Sensor/LConn1
  Electrical Reference/LConn1 -- Voltage Sensor/RConn2
  PS-Simulink Converter/LConn1 -- Voltage Sensor/RConn1

== system RAM_Design/Subsystem1/8Bit RAM 0/Subsystem9 ==
  Enable : Inport
  Data : Inport  Port=2
  Store : Inport  Port=3
  AND : Logic  IconShape=distinctive  AllPortsSameDT=off  OutDataTypeStr=boolean
  Cast To Double : DataTypeConversion  OutDataTypeStr=double  SaturateOnIntegerOverflow=off  RndMeth=Floor
  Controlled Voltage Source : fl_lib/Electrical/Electrical Sources/Controlled Voltage Source
  D Latch : simulink_extras/Flip Flops/D Latch
  Delay One Step : Delay  DelayLength=1
  Electrical Reference : fl_lib/Electrical/Electrical Elements/Electrical Reference
  Gain : Gain  Gain=5
  Simulink-PS Converter : nesl_utility/Simulink-PS Converter  PhysicalDomain=network_engine_domain  SubClassName=ps_input  LeftPortType=input  RightPortType=output  PseudoPeriodic=off  Frequencies=[]  NoiseDistribution=none  NoiseParameters=[]  Unit=1  AffineConversion=off  FilteringAndDerivatives=provide  SimscapeFilterOrder=1  InputFilterTimeConstant=0.001  UdotUserProvided=0
  Q : PMIOPort  Side=Right
  StoredVal : Outport
  wires:
  AND/1 -> Delay One Step/1
  Store/1 -> D Latch/2
  Gain/1 -> Simulink-PS Converter/1
  D Latch/1 -> StoredVal/1, AND/1
  Cast To Double/1 -> Gain/1
  Enable/1 -> AND/2
  Data/1 -> D Latch/1
  Delay One Step/1 -> Cast To Double/1
  connections:
  Controlled Voltage Source/RConn1 -- Simulink-PS Converter/RConn1
  Electrical Reference/LConn1 -- Controlled Voltage Source/RConn2
  Controlled Voltage Source/LConn1 -- Q/RConn1
